simulink model "stateflow_example_org"  (Simulink 10.0)
settings: Solver=FixedStepDiscrete  StartTime=0.0  StopTime=2200  FixedStep=1  RelTol=1e-3
libraries: simulink x1
settings Model: DataTypeOverride=Off  Creator=bsoheili  LastModifiedBy=annonymous
settings DataIOCC: LimitDataPoints=on  SaveOutput=off  SaveTime=off
settings OptimizationCC: BlockReduction=off  ConditionallyExecuteInputs=off  DefaultParameterBehavior=Inlined  UseDivisionForNetSlopeComputation=UseDivisionForReciprocalsOfIntegersOnly  UseFloatMulNetSlope=on  InlineInvariantSignals=on  EnhancedBackFolding=on  EfficientFloat2IntCast=on  LifeSpan=1  EfficientTunableParamExpr=on
settings DebuggingCC: AlgebraicLoopMsg=error  UnderspecifiedInitializationDetection=Simplified  MergeDetectMultiDrivingBlocksExec=error  InheritedTsInSrcMsg=none  SingleTaskRateTransMsg=error  AllowSymbolicDim=off  StrictBusMsg=ErrorOnBusTreatedAsVector  NonBusSignalsTreatedAsBus=error
settings HardwareCC: ProdHWDeviceType=ASIC/FPGA->ASIC/FPGA  ProdEqTarget=off
settings SFSimCC: MATLABDynamicMemAlloc=off
settings RTWCC: Description=Embedded Coder  SystemTargetFile=ert.tlc  TemplateMakefile=ert_default_tmf  GenerateReport=on  IncludeHyperlinkInReport=on  LaunchReport=on  GenerateTraceInfo=on  GenerateTraceReport=on  GenerateTraceReportSl=on  GenerateTraceReportSf=on  GenerateTraceReportEml=on  GenerateCodeMetricsReport=on
settings CodeAppCC: IgnoreCustomStorageClasses=off
settings ERTTargetCC: MultiwordLength=2048  GenerateSampleERTMain=on  CombineSignalStateStructs=on  SuppressErrorStatus=on  InlinedParameterPlacement=NonHierarchical  ERTCustomFileTemplate=example_file_process.tlc  ConvertIfToSwitch=off  SuppressUnreachableDefaultCases=off
settings ConfigComp: CovExternalEMLEnable=off

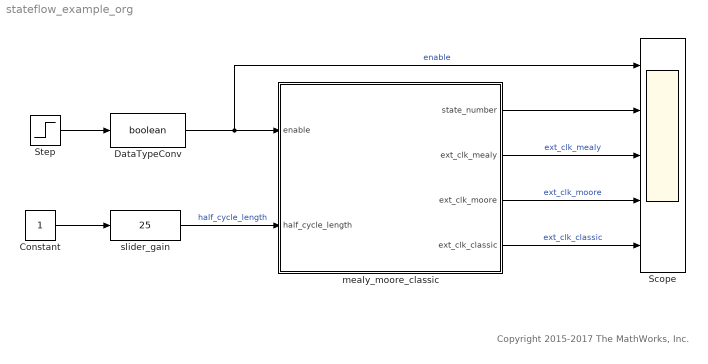
== system stateflow_example_org ==
  note: Copyright 2015-2017 The MathWorks, Inc.
  Constant : Constant  OutDataTypeStr=int16  SampleTime=1
  DataTypeConv : DataTypeConversion  OutDataTypeStr=boolean
  Scope : Scope  NumInputPorts=5
  Step : Step  Time=25  SampleTime=1
  mealy_moore_classic : Subsystem
  slider_gain : simulink/Math Operations/Slider Gain  gain=25  low=0  high=255
  wires:
  DataTypeConv/1 -> Scope/1, mealy_moore_classic/1(enable)  "enable"
  Constant/1 -> slider_gain/1
  slider_gain/1 -> mealy_moore_classic/2(half_cycle_length)  "half_cycle_length"
  Step/1 -> DataTypeConv/1
  mealy_moore_classic/1(state_number) -> Scope/2
  mealy_moore_classic/2(ext_clk_mealy) -> Scope/3  "ext_clk_mealy"
  mealy_moore_classic/3(ext_clk_moore) -> Scope/4  "ext_clk_moore"
  mealy_moore_classic/4(ext_clk_classic) -> Scope/5  "ext_clk_classic"

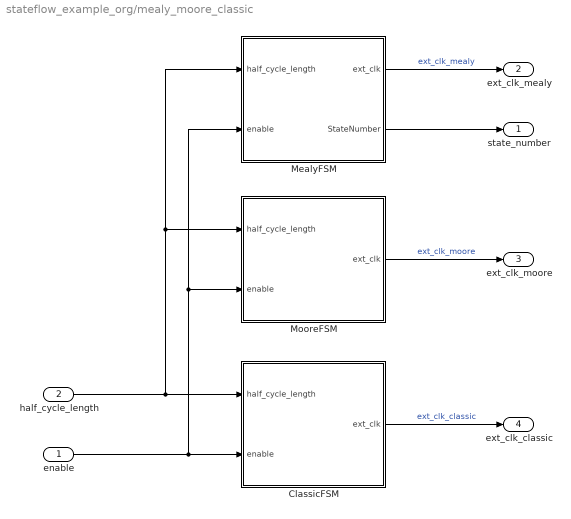
== system stateflow_example_org/mealy_moore_classic ==
  enable : Inport
  half_cycle_length : Inport  Port=2
  ClassicFSM : Subsystem
  MealyFSM : Subsystem
  MooreFSM : Subsystem
  state_number : Outport
  ext_clk_mealy : Outport  Port=2
  ext_clk_moore : Outport  Port=3
  ext_clk_classic : Outport  Port=4
  wires:
  MooreFSM/1(ext_clk) -> ext_clk_moore/1  "ext_clk_moore"
  ClassicFSM/1(ext_clk) -> ext_clk_classic/1  "ext_clk_classic"
  half_cycle_length/1 -> ClassicFSM/1(half_cycle_length), MooreFSM/1(half_cycle_length), MealyFSM/1(half_cycle_length)
  enable/1 -> ClassicFSM/2(enable), MooreFSM/2(enable), MealyFSM/2(enable)
  MealyFSM/1(ext_clk) -> ext_clk_mealy/1  "ext_clk_mealy"
  MealyFSM/2(StateNumber) -> state_number/1

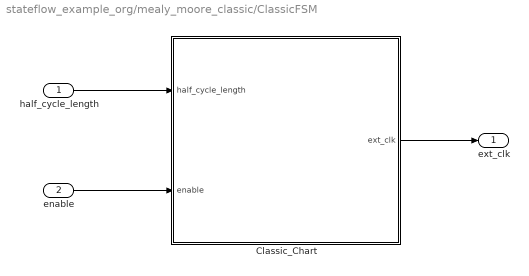
== system stateflow_example_org/mealy_moore_classic/ClassicFSM ==
  half_cycle_length : Inport
  enable : Inport  Port=2
  Classic_Chart : Stateflow chart  TreatAsAtomicUnit=on
  ext_clk : Outport
  wires:
  Classic_Chart/1(ext_clk) -> ext_clk/1
  enable/1 -> Classic_Chart/2(enable)
  half_cycle_length/1 -> Classic_Chart/1(half_cycle_length)

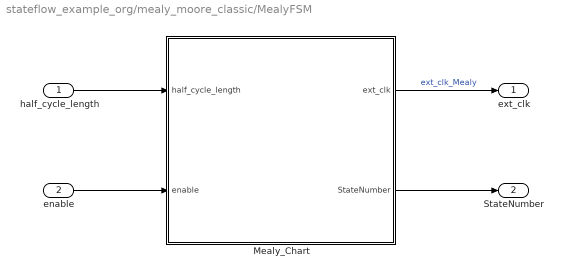
== system stateflow_example_org/mealy_moore_classic/MealyFSM ==
  half_cycle_length : Inport
  enable : Inport  Port=2
  Mealy_Chart : Stateflow chart  TreatAsAtomicUnit=on
  ext_clk : Outport
  StateNumber : Outport  Port=2
  wires:
  Mealy_Chart/1(ext_clk) -> ext_clk/1  "ext_clk_Mealy"
  half_cycle_length/1 -> Mealy_Chart/1(half_cycle_length)
  enable/1 -> Mealy_Chart/2(enable)
  Mealy_Chart/2(StateNumber) -> StateNumber/1

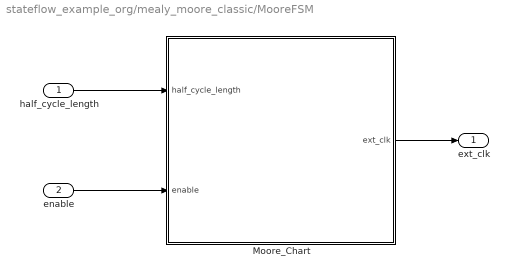
== system stateflow_example_org/mealy_moore_classic/MooreFSM ==
  half_cycle_length : Inport
  enable : Inport  Port=2
  Moore_Chart : Stateflow chart  TreatAsAtomicUnit=on
  ext_clk : Outport
  wires:
  enable/1 -> Moore_Chart/2(enable)
  Moore_Chart/1(ext_clk) -> ext_clk/1
  half_cycle_length/1 -> Moore_Chart/1(half_cycle_length)

== stateflow chart mealy_moore_classic/ClassicFSM/Classic_Chart ==
  settings: executeAtInitialization=1
  note: Note:
      | In Classic charts outputs and internal values can be generated, both, in states or during state transition.
  state s0
  state delayTime
    entry: ext_clk = false;
  state reversOutput
    entry: ext_clk = true;
  (default) -> s0 : {ext_clk = false;
      |  count = int16(0);}
  reversOutput -> s0 [order 1] : [enable == false]
      | {count(:) = 0;}
  s0 -> delayTime : [enable == true]
  delayTime -> delayTime [order 2] : {count(:) = count + 1;}
  reversOutput -> delayTime [order 2] : [count >= half_cycle_length-1]
      | {count(:) = 0;}
  delayTime -> reversOutput [order 1] : [count >= half_cycle_length-1]
      | {count(:) = 0;}
  reversOutput -> reversOutput [order 3] : {count(:) = count + 1;}
  data: half_cycle_length input int16; ext_clk output boolean; enable input boolean; count local int16

== stateflow chart mealy_moore_classic/MealyFSM/Mealy_Chart ==
  settings: stateMachineType=MEALY_MACHINE  executeAtInitialization=1
  note: Note:
      | Outputs and internal values are generated during the state transition in Mealy Machines.
  state idle
  state delayTime
  state reversOutput
  (default) -> idle : {ext_clk = false;
      |  count = int16(0);}
  reversOutput -> idle [order 1] : [enable == false]
      | {ext_clk = false;}
  idle -> delayTime : [enable == true]
      | {ext_clk = false;}
  delayTime -> delayTime [order 2] : {count(:) = count + 1;}
  reversOutput -> delayTime [order 2] : [count >= half_cycle_length-1]
      | {ext_clk = false;
      | count(:) = 0;}
  delayTime -> reversOutput [order 1] : [count >= half_cycle_length -1]
      | {ext_clk = true;
      | count(:) = 0;}
  reversOutput -> reversOutput [order 3] : {count(:) = count + 1;}
  data: half_cycle_length input int16; ext_clk output boolean; enable input boolean; count local int16; StateNumber output Enum: MealyChartNumber

== stateflow chart mealy_moore_classic/MooreFSM/Moore_Chart ==
  settings: stateMachineType=MOORE_MACHINE  executeAtInitialization=1  initializeOutput=1
  note: Note:
      | In Moore machines the outputs and internal values (such as internal_cntr in this example) are updated only inside the states. Because of this Moore machines usually require more states and therefore also use more resources.
  state idle
    ext_clk = false;
    internal_cntr = int16(0);
  state delayTime1
    ext_clk = false;
    internal_cntr(:) = internal_cntr + 1;
  state reverseOutput2
    ext_clk = false;
    internal_cntr(:) = 0;
  state reverseOutput1
    ext_clk = true;
    internal_cntr(:) = 0;
  state delayTime2
    ext_clk = true;
    internal_cntr(:) = internal_cntr + 1;
  (default) -> idle
  reverseOutput1 -> idle [order 1] : [enable == false]
  idle -> delayTime1 : [enable == true]
  reverseOutput2 -> delayTime1
  delayTime1 -> reverseOutput1 : [internal_cntr >= half_cycle_length-1]
  delayTime2 -> reverseOutput2 : [internal_cntr >= half_cycle_length-1]
  reverseOutput1 -> delayTime2 [order 2]
  data: half_cycle_length input int16; enable input boolean; internal_cntr local int16; ext_clk output boolean
